simulink model "PID_Heizung"  (R2013b)
settings: Solver=ode1  StartTime=0.0  StopTime=100  FixedStep=dT  RelTol=1e-3
undefined symbols (not defined in the file): c1, c2, I, P, Theta_A, Theta_offset, Theta_s
libraries: simulink x1
settings Model: Creator=daltdoer  LastModifiedBy=daltdoer

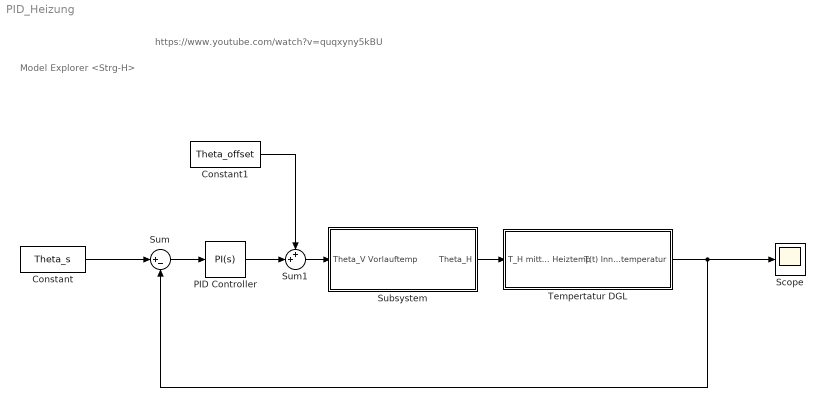
== system PID_Heizung ==
  note: Model Explorer <Strg-H>
  note: https://www.youtube.com/watch?v=quqxyny5kBU
  Constant : Constant  Value=Theta_s
  Constant1 : Constant  Value=Theta_offset
  PID Controller : simulink/Continuous/PID Controller  Controller=PI  TimeDomain=Continuous-time  SampleTime=1  IntegratorMethod=Forward Euler  FilterMethod=Forward Euler  Form=Ideal  P=P  I=I  D=0  N=100  InitialConditionSource=internal  InitialConditionForIntegrator=0  InitialConditionForFilter=0  ExternalReset=none  LimitOutput=off  UpperSaturationLimit=inf  LowerSaturationLimit=-inf  LinearizeAsGain=on  AntiWindupMode=none  Kb=1  TrackingMode=off  Kt=1  PParamMin=[]  PParamMax=[]  IParamMin=[]  IParamMax=[]  DParamMin=[]  DParamMax=[]  NParamMin=[]  NParamMax=[]  KbParamMin=[]  KbParamMax=[]  KtParamMin=[]  KtParamMax=[]  POutMin=[]  POutMax=[]  IOutMin=[]  IOutMax=[]  DOutMin=[]  DOutMax=[]  NOutMin=[]  NOutMax=[]  KbOutMin=[]  KbOutMax=[]  KtOutMin=[]  KtOutMax=[]  IntegratorOutMin=[]  IntegratorOutMax=[]  FilterOutMin=[]  FilterOutMax=[]  SumOutMin=[]  SumOutMax=[]  SumI1OutMin=[]  SumI1OutMax=[]  SumI2OutMin=[]  SumI2OutMax=[]  SumI3OutMin=[]  SumI3OutMax=[]  SumDOutMin=[]  SumDOutMax=[]  SaturationOutMin=[]  SaturationOutMax=[]  IntegratorContinuousStateAttributes=''  IntegratorStateMustResolveToSignalObject=off  IntegratorRTWStateStorageClass=Auto  FilterContinuousStateAttributes=''  FilterStateMustResolveToSignalObject=off  FilterRTWStateStorageClass=Auto
  Scope : Scope
  Subsystem : Subsystem
  Sum : Sum  Inputs=|+-
  Sum1 : Sum  Inputs=++|
  "Tempertatur DGL " : Subsystem
  wires:
  Constant/1 -> Sum/1
  Sum/1 -> PID Controller/1
  "Tempertatur DGL "/1(T(t) Innentemperatur) -> Scope/1, Sum/2
  Subsystem/1(Theta_H) -> "Tempertatur DGL "/1("T_H mittlere Heiztemp ")
  PID Controller/1 -> Sum1/2
  Sum1/1 -> Subsystem/1(Theta_V Vorlauftemp)
  Constant1/1 -> Sum1/1

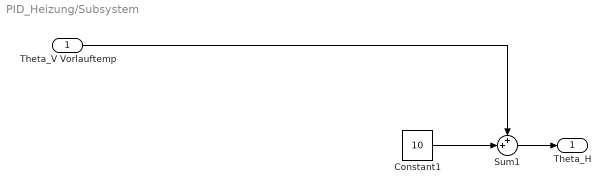
== system PID_Heizung/Subsystem ==
  Theta_V Vorlauftemp : Inport
  Constant1 : Constant  Value=10
  Sum1 : Sum  Inputs=++|
  Theta_H : Outport
  wires:
  Theta_V Vorlauftemp/1 -> Sum1/1
  Constant1/1 -> Sum1/2
  Sum1/1 -> Theta_H/1

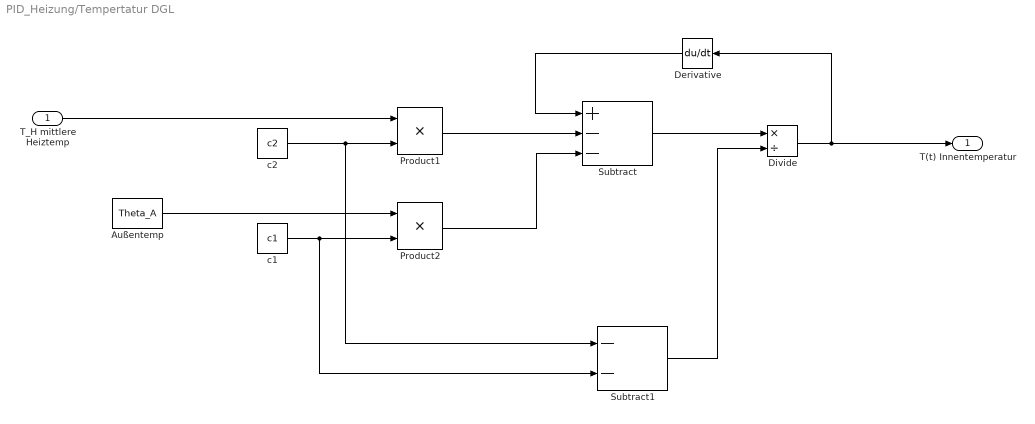
== system PID_Heizung/Tempertatur DGL  ==
  "T_H mittlere Heiztemp " : Inport
  Außentemp : Constant  Value=Theta_A
  Derivative : Derivative
  Divide : Product  Inputs=*/
  Product1 : Product
  Product2 : Product
  Subtract : Sum  Inputs=+--
  Subtract1 : Sum  Inputs=--
  c1 : Constant  Value=c1
  c2 : Constant  Value=c2
  T(t) Innentemperatur : Outport
  wires:
  Divide/1 -> T(t) Innentemperatur/1, Derivative/1
  Außentemp/1 -> Product2/1
  c1/1 -> Subtract1/2, Product2/2
  "T_H mittlere Heiztemp "/1 -> Product1/1
  c2/1 -> Subtract1/1, Product1/2
  Derivative/1 -> Subtract/1
  Product1/1 -> Subtract/2
  Product2/1 -> Subtract/3
  Subtract/1 -> Divide/1
  Subtract1/1 -> Divide/2
